simulink model "simu"  (R2018b)
settings: Solver=VariableStepAuto  StartTime=0.0  StopTime=10.0e-3  RelTol=1e-3
values from neighbouring files (symbols this model uses):
  Ts = t(2)-t(1)    [freq_analysis.m]    (also in simulink_vars.m = 0.002; step_analysis.m = 5e-05; step_analysis_pos.m = 0.02)
libraries: simulink x4
settings Model: Creator=javi  LastModifiedBy=javi

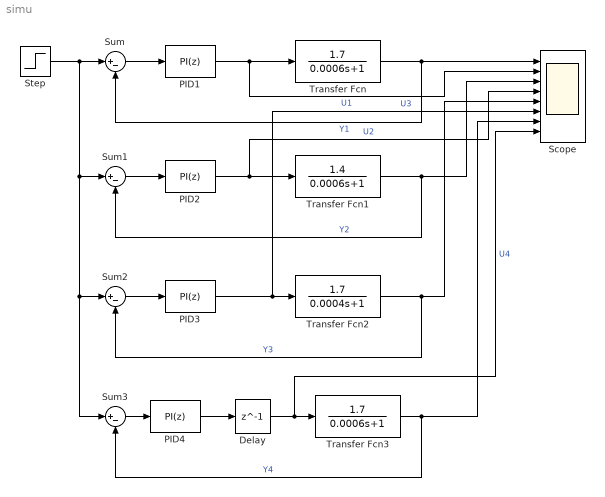
== system simu ==
  Delay : Delay  DelayLength=1
  PID{1..4} (4 alike) : simulink/Continuous/PID Controller  Controller=PI  Form=Parallel  TimeDomain=Discrete-time  SampleTime=Ts  IntegratorMethod=Forward Euler  FilterMethod=Forward Euler  ControllerParametersSource=internal  P=0.8  I=3075  D=0  UseFilter=on  N=100  TunerSelectOption=Transfer Function Based (PID Tuner App)  InitialConditionSource=internal  InitialConditionForIntegrator=0  InitialConditionForFilter=0  DifferentiatorICPrevScaledInput=0  ExternalReset=none  TrackingMode=off  Kt=1  LimitOutput=on  UpperSaturationLimit=1800  LowerSaturationLimit=0  LinearizeAsGain=off  AntiWindupMode=clamping  Kb=1  POutMin=[]  POutMax=[]  IOutMin=[]  IOutMax=[]  DOutMin=[]  DOutMax=[]  NOutMin=[]  NOutMax=[]  SumOutMin=[]  SumOutMax=[]  SaturationOutMin=[]  SaturationOutMax=[]  PParamMin=[]  PParamMax=[]  IParamMin=[]  IParamMax=[]  DParamMin=[]  DParamMax=[]  NParamMin=[]  NParamMax=[]  KbParamMin=[]  KbParamMax=[]  KtParamMin=[]  KtParamMax=[]  KbOutMin=[]  KbOutMax=[]  KtOutMin=[]  KtOutMax=[]  IntegratorOutMin=[]  IntegratorOutMax=[]  FilterOutMin=[]  FilterOutMax=[]  SumI1OutMin=[]  SumI1OutMax=[]  SumI2OutMin=[]  SumI2OutMax=[]  SumI3OutMin=[]  SumI3OutMax=[]  SumI4OutMin=[]  SumI4OutMax=[]  SumDOutMin=[]  SumDOutMax=[]  DifferentiatorOutMin=[]  DifferentiatorOutMax=[]  FilterDiffOutCoefMin=[]  FilterDiffOutCoefMax=[]  ReciprocalOutMin=[]  ReciprocalOutMax=[]  SumDenOutMin=[]  SumDenOutMax=[]  SumNumOutMin=[]  SumNumOutMax=[]  DivideOutMin=[]  DivideOutMax=[]  IntegratorContinuousStateAttributes=''  IntegratorStateMustResolveToSignalObject=off  IntegratorRTWStateStorageClass=Auto  FilterContinuousStateAttributes=''  FilterStateMustResolveToSignalObject=off  FilterRTWStateStorageClass=Auto  ParallelPVariant=InternalParameters  IdealPVariant=Disabled  IVariant=InternalParameters  DVariant=Disabled  IntegratorVariant=Discrete  SatVariant=Enabled  AWVariant=DiscClampingParallel  PCopyVariant=Disabled  TRVariant=Disabled  FdbkBlocksVariant=Forward  IdealPFdbkVariant=Disabled  SatFdbkVariant=Disabled  DerivativeFilterVariant=Disabled  NVariant=Disabled  NCopyVariant=Disabled_SignalSpec  FilterICVariant=Disabled  IntegratorICVariant=InternalICs  ExternalResetVariant=Disabled  TRSumVariant=Passthrough  SumFdbkVariant=Disabled  SumVariant=Sum_PI
  Scope : Scope  NumInputPorts=8
  Step : Step  Time=0  After=1500  SampleTime=Ts
  Sum{,1..3} (4 alike) : Sum  Inputs=|+-
  Transfer Fcn : TransferFcn  Numerator=[1.7]  Denominator=[0.0006 1]
  Transfer Fcn1 : TransferFcn  Numerator=[1.4]  Denominator=[0.0006 1]
  Transfer Fcn2 : TransferFcn  Numerator=[1.7]  Denominator=[0.0004 1]
  Transfer Fcn3 : TransferFcn  Numerator=[1.7]  Denominator=[0.0006 1]
  wires:
  Transfer Fcn/1 -> Sum/2, Scope/1  "Y1"
  PID1/1 -> Scope/2, Transfer Fcn/1  "U1"
  Sum/1 -> PID1/1
  PID2/1 -> Scope/4, Transfer Fcn1/1  "U2"
  Sum1/1 -> PID2/1
  Transfer Fcn1/1 -> Scope/3, Sum1/2  "Y2"
  PID3/1 -> Scope/6, Transfer Fcn2/1  "U3"
  Sum2/1 -> PID3/1
  Transfer Fcn2/1 -> Scope/5, Sum2/2  "Y3"
  PID4/1 -> Delay/1
  Transfer Fcn3/1 -> Scope/7, Sum3/2  "Y4"
  Step/1 -> Sum3/1, Sum2/1, Sum1/1, Sum/1
  Sum3/1 -> PID4/1
  Delay/1 -> Scope/8, Transfer Fcn3/1  "U4"
